simulink model "toplevel"  (R2015a)
settings: Solver=FixedStepDiscrete  StartTime=0.0  StopTime=1.0  FixedStep=0.01  RelTol=1e-3
libraries: IGStatus x1
settings Model: Creator=mbd_user  LastModifiedBy=mbd_user
settings HardwareCC: ProdIntDivRoundTo=Zero

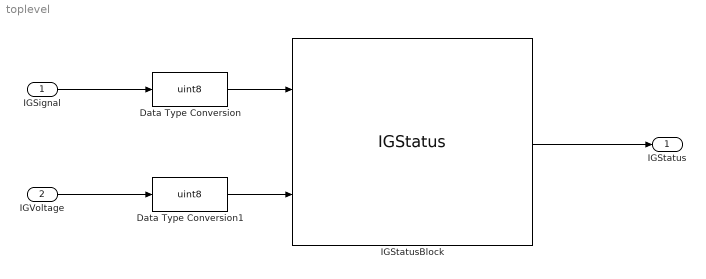
== system toplevel ==
  IGSignal : Inport
  IGVoltage : Inport  Port=2
  Data Type Conversion : DataTypeConversion  OutDataTypeStr=uint8
  Data Type Conversion1 : DataTypeConversion  OutDataTypeStr=uint8
  IGStatusBlock : IGStatus/IGStatus
  IGStatus : Outport
  wires:
  IGStatusBlock/1 -> IGStatus/1
  Data Type Conversion/1 -> IGStatusBlock/1
  IGSignal/1 -> Data Type Conversion/1
  IGVoltage/1 -> Data Type Conversion1/1
  Data Type Conversion1/1 -> IGStatusBlock/2
